simulink model "VDSAFARI"  (R2020b)
settings: Solver=VariableStepAuto  StartTime=0.0  StopTime=8.85  RelTol=1e-3
values from neighbouring files (symbols this model uses):
  AirDensity = 1.2256    [VDSUVSimlink.m]    (also in VDSafari.m)
  AirDragCoefficient = 0.45    [VDSUVSimlink.m]    (also in VDSafari.m)
  AllowedFrontLoad = 500 * g    (= 4900)    [VDSUVSimlink.m]    (also in VDSafari.m)
  CarWeight = KerbWeight + DriverWeight    (= 1745)    [VDSUVSimlink.m]    (also in VDSafari.m)
  CoefficientOfFriction = 0.9    [VDSUVSimlink.m]    (also in VDSafari.m)
  CoefficientOfRollingResistance = 0.035    [VDSUVSimlink.m]    (also in VDSafari.m)
  Equation = polyfit(EngineRadPs,EngineTorque,2)    [VDSUVSimlink.m]    (also in VDSafari.m)
  FinalDrive = 3.75    [VDSUVSimlink.m]    (also in VDSafari.m)
  FrontalArea = 3.138    [VDSUVSimlink.m]    (also in VDSafari.m)
  FrontWheelRadius = 0.369    [VDSUVSimlink.m]    (also in VDSafari.m)
  g = 9.8    [VDSUVSimlink.m]    (also in VDSafari.m)
  GearNo = Gears(1,1)    [VDSUVSimlink.m]    (also in VDSafari.m = 6)
  Gears = [1 3.96 ; 2 2.210 ; 3 1.422 ; 4 1 ; 5 0.779 ; 6 0.710]    [VDSUVSimlink.m]    (also in VDSafari.m)
  Height = 0.800    (= 0.8)    [VDSUVSimlink.m]    (also in VDSafari.m)
  MaximumEngineRPM = 3600    [VDSUVSimlink.m]    (also in VDSafari.m)
  MaximumGears = 6    [VDSUVSimlink.m]    (also in VDSafari.m)
  MinimumEngineRPM = 1200    [VDSUVSimlink.m]    (also in VDSafari.m)
  StaticFrontLoad = 0.64 *CarWeight*g    (= 10944.64)    [VDSUVSimlink.m]    (also in VDSafari.m)
  Wheelbase = 2.741    [VDSUVSimlink.m]    (also in VDSafari.m)
libraries: simulink x1
settings Model: Creator=dinesh  LastModifiedBy=dinesh

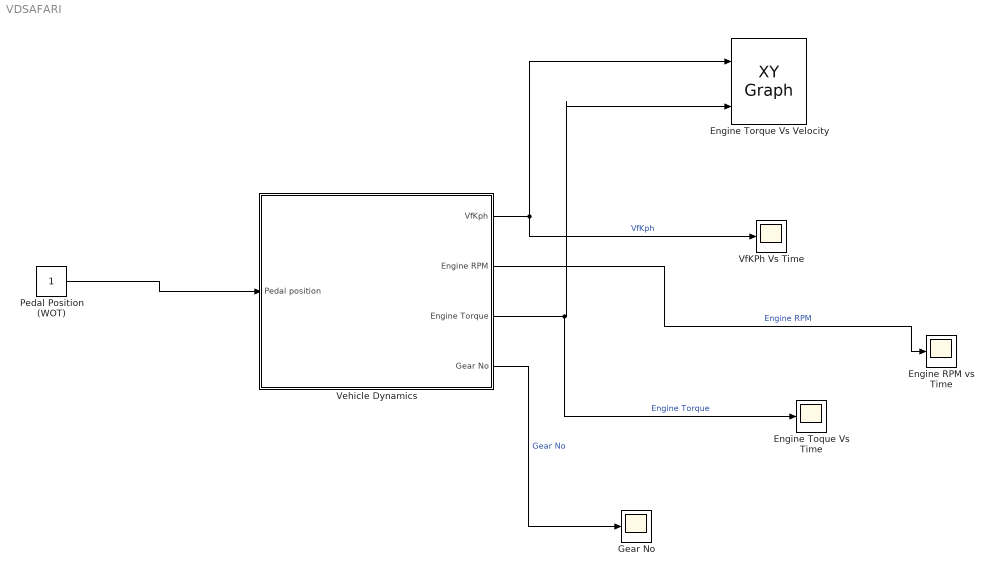
== system VDSAFARI ==
  Engine RPM vs Time : Scope
  Engine Toque Vs Time : Scope
  Engine Torque Vs Velocity : simulink/Sinks/XY Graph  xmin=0  xmax=150  ymin=0  ymax=400  st=-1
  Gear No : Scope
  Pedal Position (WOT) : Constant
  Vehicle Dynamics : Subsystem
  VfKPh Vs Time : Scope
  wires:
  Pedal Position (WOT)/1 -> Vehicle Dynamics/1(Pedal position)
  Vehicle Dynamics/3(Engine Torque) -> Engine Toque Vs Time/1, Engine Torque Vs Velocity/2  "Engine Torque"
  Vehicle Dynamics/1(VfKph) -> VfKPh Vs Time/1, Engine Torque Vs Velocity/1  "VfKph"
  Vehicle Dynamics/4(Gear No) -> Gear No/1  "Gear No"
  Vehicle Dynamics/2(Engine RPM) -> Engine RPM vs Time/1  "Engine RPM"

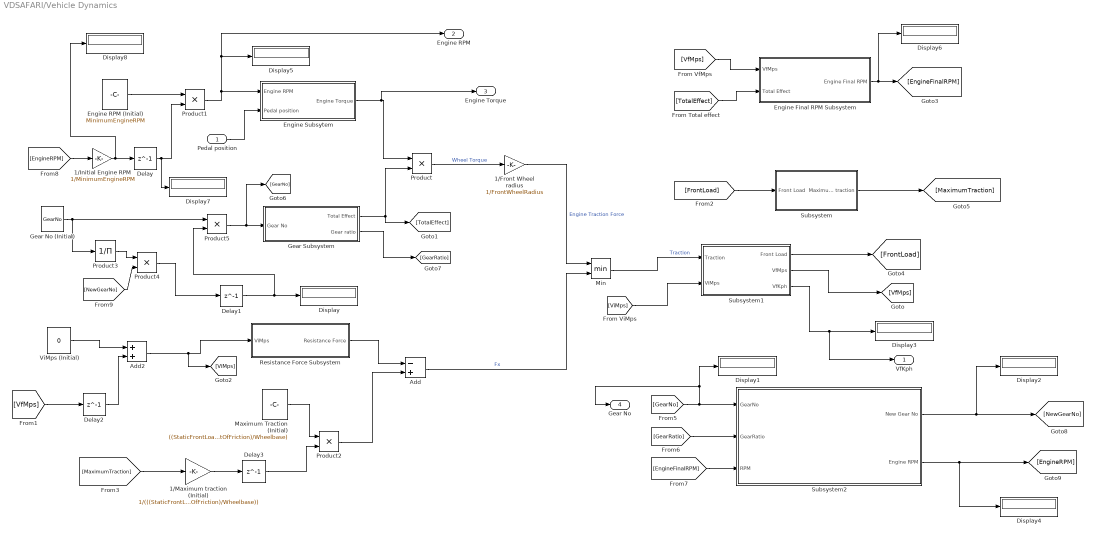
== system VDSAFARI/Vehicle Dynamics ==
  Pedal position : Inport
  1/Front Wheel radius : Gain  Gain=1/FrontWheelRadius
  1/Initial Engine RPM : Gain  Gain=1/MinimumEngineRPM
  1/Maximum traction (Initial) : Gain  Gain=1/(((StaticFrontLoad*CoefficientOfFriction))/(1+(Height*CoefficientOfFriction)/Wheelbase))
  Add : Sum  Inputs=-+
  Add2 : Sum
  Delay : Delay  DelayLength=1  InitialCondition=1  SampleTime=0.001
  Delay1 : Delay  DelayLength=1  InitialCondition=1  SampleTime=0.001
  Delay2 : Delay  DelayLength=1  InitialCondition=0  SampleTime=0.001
  Delay3 : Delay  DelayLength=1  InitialCondition=1  SampleTime=0.001
  Display{,1..8} (9 alike) : Display
  Engine Final RPM Subsystem : Subsystem
  Engine RPM (Initial) : Constant  Value=MinimumEngineRPM
  Engine Subsytem : Subsystem
  Gear No (Initial) : Constant  Value=GearNo
  Gear Subsystem : Subsystem
  Maximum Traction (Initial) : Constant  Value=((StaticFrontLoad*CoefficientOfFriction))/(1+(Height*CoefficientOfFriction)/Wheelbase)
  Min : MinMax  Inputs=2
  Product{,1..2,4..5} (5 alike) : Product
  Product3 : Product  Inputs=/
  Resistance Force Subsystem : Subsystem
  Subsystem : Subsystem
  Subsystem1 : Subsystem
  Subsystem2 : Subsystem
  ViMps (Initial) : Constant  Value=0
  VfKph : Outport
  Engine RPM : Outport  Port=2
  Engine Torque : Outport  Port=3
  Gear No : Outport  Port=4
  wires:
  Resistance Force Subsystem/1(Resistance Force) -> Add/1
  Add/1 -> Min/2  "Fx"
  Gear No (Initial)/1 -> Product5/1, Product3/1
  Engine Subsytem/1(Engine Torque) -> Engine Torque/1, Product/1
  Gear Subsystem/1(Total Effect) -> [TotalEffect], Product/2
  Product/1 -> 1/Front Wheel radius/1  "Wheel Torque"
  1/Front Wheel radius/1 -> Min/1  "Engine Traction Force"
  [TotalEffect] -> Engine Final RPM Subsystem/2(Total Effect)
  [VfMps] -> Engine Final RPM Subsystem/1(VfMps)
  Engine Final RPM Subsystem/1(Engine Final RPM) -> Display6/1, [EngineFinalRPM]
  [EngineRPM] -> 1/Initial Engine RPM/1
  1/Initial Engine RPM/1 -> Delay/1, Display8/1
  Engine RPM (Initial)/1 -> Product1/1
  Delay/1 -> Display7/1, Product1/2
  Product1/1 -> Engine RPM/1, Display5/1, Engine Subsytem/1(Engine RPM)
  [VfMps] -> Delay2/1
  ViMps (Initial)/1 -> Add2/1
  Delay2/1 -> Add2/2
  Add2/1 -> [ViMps], Resistance Force Subsystem/1(ViMps)
  [FrontLoad] -> Subsystem/1(Front Load)
  Subsystem/1(Maximum traction) -> [MaximumTraction]
  Maximum Traction (Initial)/1 -> Product2/1
  [MaximumTraction] -> 1/Maximum traction (Initial)/1
  1/Maximum traction (Initial)/1 -> Delay3/1
  Delay3/1 -> Product2/2
  Product2/1 -> Add/2
  Min/1 -> Subsystem1/1(Traction)  "Traction"
  Subsystem1/1(Front Load) -> [FrontLoad]
  Subsystem1/2(VfMps) -> [VfMps]
  Subsystem1/3(VfKph) -> VfKph/1, Display3/1
  [ViMps] -> Subsystem1/2(ViMps)
  Pedal position/1 -> Engine Subsytem/2(Pedal position)
  Gear Subsystem/2(Gear ratio) -> [GearRatio]
  Product3/1 -> Product4/1
  [NewGearNo] -> Product4/2
  Product4/1 -> Delay1/1
  Product5/1 -> [GearNo], Gear Subsystem/1(Gear No)
  [GearNo] -> Display1/1, Gear No/1, Subsystem2/1(GearNo)
  [GearRatio] -> Subsystem2/2(GearRatio)
  [EngineFinalRPM] -> Subsystem2/3(" RPM")
  Subsystem2/1(New Gear No) -> Display2/1, [NewGearNo]
  Subsystem2/2(Engine RPM) -> Display4/1, [EngineRPM]
  Delay1/1 -> Product5/2, Display/1

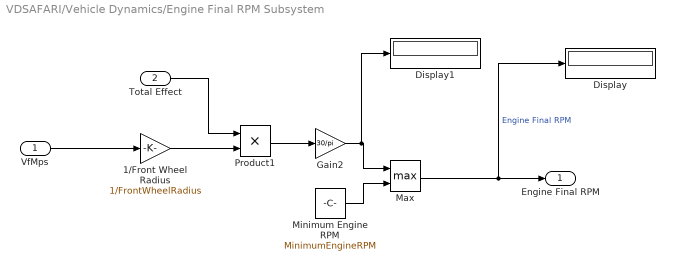
== system VDSAFARI/Vehicle Dynamics/Engine Final RPM Subsystem ==
  VfMps : Inport
  Total Effect : Inport  Port=2
  1/Front Wheel Radius : Gain  Gain=1/FrontWheelRadius
  Display : Display
  Display1 : Display
  Gain2 : Gain  Gain=30/pi
  Max : MinMax  Function=max  Inputs=2
  Minimum Engine RPM : Constant  Value=MinimumEngineRPM
  Product1 : Product
  Engine Final RPM : Outport
  wires:
  Gain2/1 -> Display1/1, Max/1
  Minimum Engine RPM/1 -> Max/2
  Max/1 -> Display/1, Engine Final RPM/1  "Engine Final RPM"
  1/Front Wheel Radius/1 -> Product1/2
  Product1/1 -> Gain2/1
  VfMps/1 -> 1/Front Wheel Radius/1
  Total Effect/1 -> Product1/1

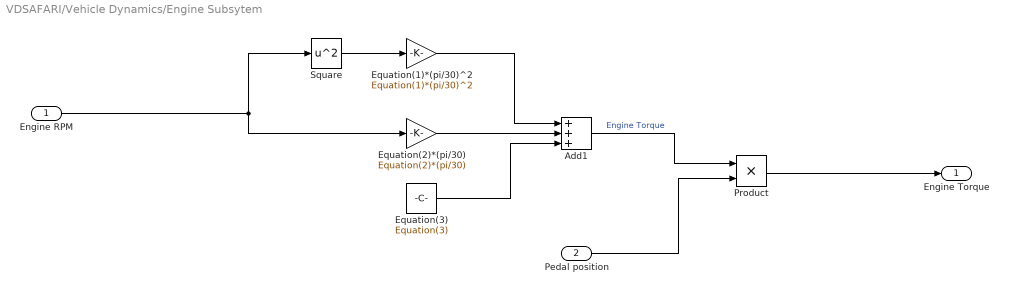
== system VDSAFARI/Vehicle Dynamics/Engine Subsytem ==
  Engine RPM : Inport
  Pedal position : Inport  Port=2
  Add1 : Sum  Inputs=+++
  "Equation(1)*(pi/30)^2 " : Gain  Gain=Equation(1)*(pi/30)^2
  Equation(2)*(pi/30) : Gain  Gain=Equation(2)*(pi/30)
  Equation(3) : Constant  Value=Equation(3)
  Product : Product
  Square : Math  Operator=square  SaturateOnIntegerOverflow=on
  Engine Torque : Outport
  wires:
  Equation(2)*(pi/30)/1 -> Add1/2
  Equation(3)/1 -> Add1/3
  Square/1 -> "Equation(1)*(pi/30)^2 "/1
  "Equation(1)*(pi/30)^2 "/1 -> Add1/1
  Engine RPM/1 -> Square/1, Equation(2)*(pi/30)/1
  Add1/1 -> Product/1  "Engine Torque"
  Pedal position/1 -> Product/2
  Product/1 -> Engine Torque/1

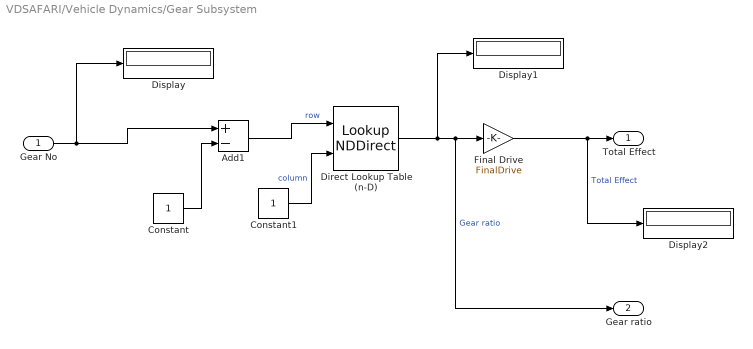
== system VDSAFARI/Vehicle Dynamics/Gear Subsystem ==
  Gear No : Inport
  Add1 : Sum  Inputs=+-
  Constant : Constant
  Constant1 : Constant
  Direct Lookup Table (n-D) : LookupNDDirect  Table=Gears  DiagnosticForOutOfRangeInput=Error
  Display : Display
  Display1 : Display
  Display2 : Display
  Final Drive : Gain  Gain=FinalDrive
  Total Effect : Outport
  Gear ratio : Outport  Port=2
  wires:
  Add1/1 -> Direct Lookup Table (n-D)/1  "row"
  Direct Lookup Table (n-D)/1 -> Display1/1, Gear ratio/1, Final Drive/1  "Gear ratio"
  Constant1/1 -> Direct Lookup Table (n-D)/2  "column"
  Constant/1 -> Add1/2
  Final Drive/1 -> Display2/1, Total Effect/1  "Total Effect"
  Gear No/1 -> Display/1, Add1/1

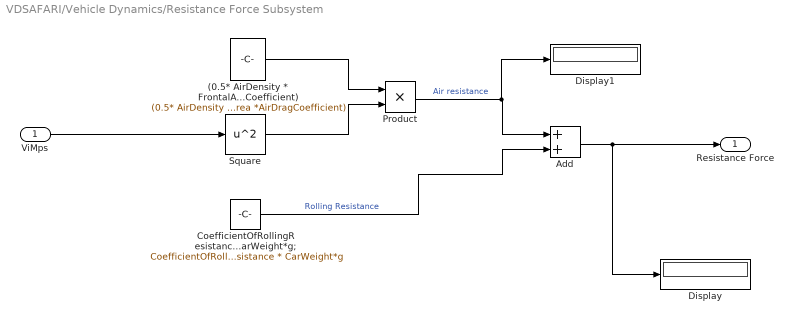
== system VDSAFARI/Vehicle Dynamics/Resistance Force Subsystem ==
  ViMps : Inport
  (0.5* AirDensity * FrontalArea * AirDragCoefficient) : Constant  Value=(0.5* AirDensity * FrontalArea *AirDragCoefficient)
  Add : Sum
  CoefficientOfRollingResistance * CarWeight*g; : Constant  Value=CoefficientOfRollingResistance * CarWeight*g
  Display : Display
  Display1 : Display
  Product : Product
  Square : Math  Operator=square  SaturateOnIntegerOverflow=on
  Resistance Force : Outport
  wires:
  Product/1 -> Display1/1, Add/1  "Air resistance"
  Add/1 -> Display/1, Resistance Force/1
  (0.5* AirDensity * FrontalArea * AirDragCoefficient)/1 -> Product/1
  Square/1 -> Product/2
  ViMps/1 -> Square/1
  CoefficientOfRollingResistance * CarWeight*g;/1 -> Add/2  "Rolling Resistance"

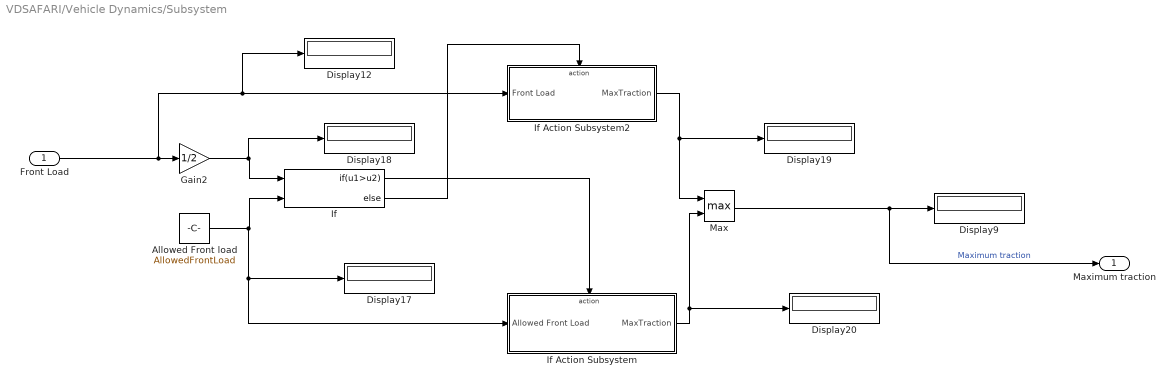
== system VDSAFARI/Vehicle Dynamics/Subsystem ==
  Front Load : Inport
  Allowed Front load : Constant  Value=AllowedFrontLoad
  Display{9,12,17..20} (6 alike) : Display
  Gain2 : Gain  Gain=1/2
  If : If  NumInputs=2  IfExpression=u1>u2
  If Action Subsystem : Subsystem  TreatAsAtomicUnit=on
  If Action Subsystem2 : Subsystem  TreatAsAtomicUnit=on
  Max : MinMax  Function=max  Inputs=2
  Maximum traction : Outport
  wires:
  If/1 -> If Action Subsystem/Action
  If/2 -> If Action Subsystem2/Action
  If Action Subsystem2/1(MaxTraction) -> Display19/1, Max/1
  Max/1 -> Maximum traction/1, Display9/1  "Maximum traction"
  Front Load/1 -> Display12/1, If Action Subsystem2/1(Front Load), Gain2/1
  Allowed Front load/1 -> Display17/1, If Action Subsystem/1(Allowed Front Load), If/2
  If Action Subsystem/1(MaxTraction) -> Max/2, Display20/1
  Gain2/1 -> Display18/1, If/1

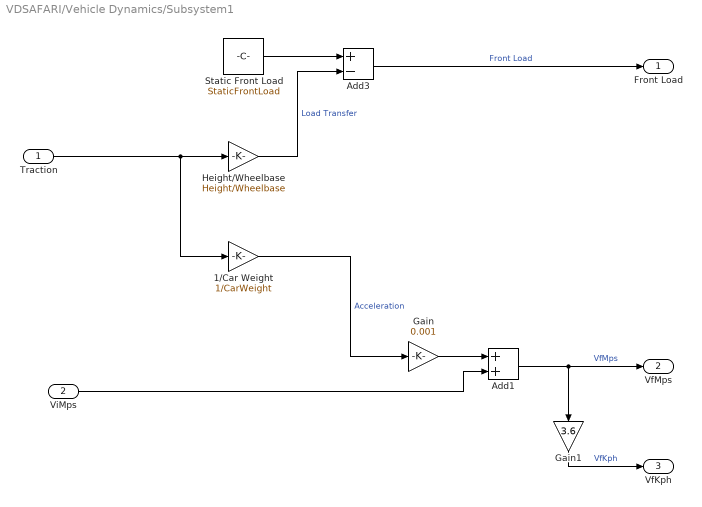
== system VDSAFARI/Vehicle Dynamics/Subsystem1 ==
  Traction : Inport
  ViMps : Inport  Port=2
  1/Car Weight : Gain  Gain=1/CarWeight
  Add1 : Sum
  Add3 : Sum  Inputs=+-
  Gain : Gain  Gain=0.001
  Gain1 : Gain  Gain=3.6
  Height/Wheelbase : Gain  Gain=Height/Wheelbase
  Static Front Load : Constant  Value=StaticFrontLoad
  Front Load : Outport
  VfMps : Outport  Port=2
  VfKph : Outport  Port=3
  wires:
  Height/Wheelbase/1 -> Add3/2  "Load Transfer"
  Gain1/1 -> VfKph/1  "VfKph"
  Add1/1 -> VfMps/1, Gain1/1  "VfMps"
  Add3/1 -> Front Load/1  "Front Load"
  Static Front Load/1 -> Add3/1
  Traction/1 -> 1/Car Weight/1, Height/Wheelbase/1
  Gain/1 -> Add1/1
  1/Car Weight/1 -> Gain/1  "Acceleration"
  ViMps/1 -> Add1/2

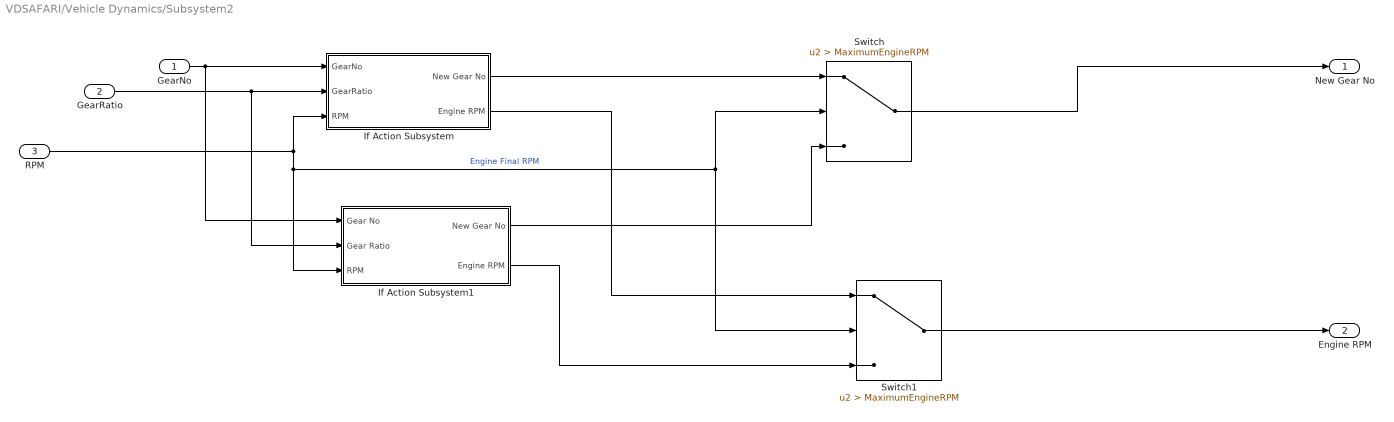
== system VDSAFARI/Vehicle Dynamics/Subsystem2 ==
  GearNo : Inport
  GearRatio : Inport  Port=2
  " RPM" : Inport  Port=3
  If Action Subsystem : Subsystem  TreatAsAtomicUnit=on
  If Action Subsystem1 : Subsystem  TreatAsAtomicUnit=on
  Switch : Switch  Criteria=u2 > Threshold  Threshold=MaximumEngineRPM
  Switch1 : Switch  Criteria=u2 > Threshold  Threshold=MaximumEngineRPM
  New Gear No : Outport
  Engine RPM : Outport  Port=2
  wires:
  If Action Subsystem1/1(New Gear No) -> Switch/3
  Switch1/1 -> Engine RPM/1
  Switch/1 -> New Gear No/1
  " RPM"/1 -> Switch/2, Switch1/2, If Action Subsystem1/3(RPM), If Action Subsystem/3(" RPM")  "Engine Final RPM"
  If Action Subsystem/1(New Gear No) -> Switch/1
  GearNo/1 -> If Action Subsystem1/1(Gear No), If Action Subsystem/1(GearNo)
  GearRatio/1 -> If Action Subsystem1/2(Gear Ratio), If Action Subsystem/2(GearRatio)
  If Action Subsystem/2(Engine RPM) -> Switch1/1
  If Action Subsystem1/2(Engine RPM) -> Switch1/3

== system VDSAFARI/Vehicle Dynamics/Subsystem/If Action Subsystem ==
  Allowed Front Load : Inport
  Action Port : ActionPort  ActionPortLabel=if(u1>u2)
  Gain : Gain  Gain=2
  mu : Gain  Gain=CoefficientOfFriction
  MaxTraction : Outport
  wires:
  Allowed Front Load/1 -> Gain/1
  Gain/1 -> mu/1
  mu/1 -> MaxTraction/1

== system VDSAFARI/Vehicle Dynamics/Subsystem/If Action Subsystem2 ==
  Front Load : Inport
  Action Port : ActionPort  ActionPortLabel=else
  Display : Display
  Display1 : Display
  mu : Gain  Gain=CoefficientOfFriction
  MaxTraction : Outport
  wires:
  Front Load/1 -> Display/1, mu/1
  mu/1 -> Display1/1, MaxTraction/1

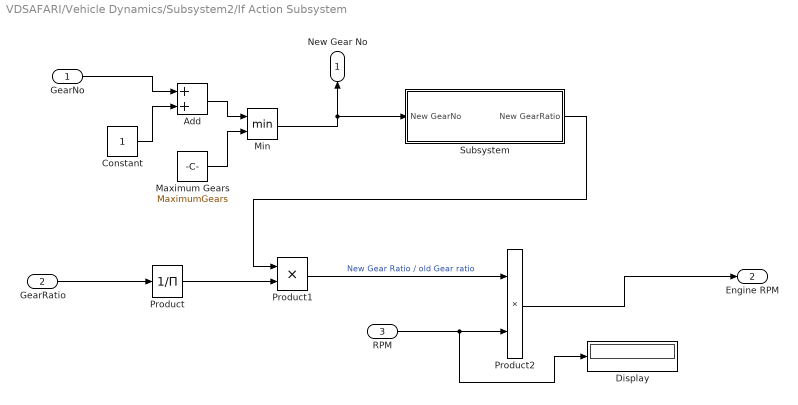
== system VDSAFARI/Vehicle Dynamics/Subsystem2/If Action Subsystem ==
  GearNo : Inport
  GearRatio : Inport  Port=2
  " RPM" : Inport  Port=3
  Add : Sum
  Constant : Constant
  Display : Display
  Maximum Gears : Constant  Value=MaximumGears
  Min : MinMax  Inputs=2
  Product : Product  Inputs=/
  Product1 : Product
  Product2 : Product
  Subsystem : Subsystem
  New Gear No : Outport
  Engine RPM : Outport  Port=2
  wires:
  GearNo/1 -> Add/1
  Constant/1 -> Add/2
  Add/1 -> Min/1
  Maximum Gears/1 -> Min/2
  Min/1 -> New Gear No/1, Subsystem/1(New GearNo)
  GearRatio/1 -> Product/1
  Product/1 -> Product1/2
  Subsystem/1(New GearRatio) -> Product1/1
  " RPM"/1 -> Display/1, Product2/2
  Product1/1 -> Product2/1  "New Gear Ratio / old Gear ratio"
  Product2/1 -> Engine RPM/1

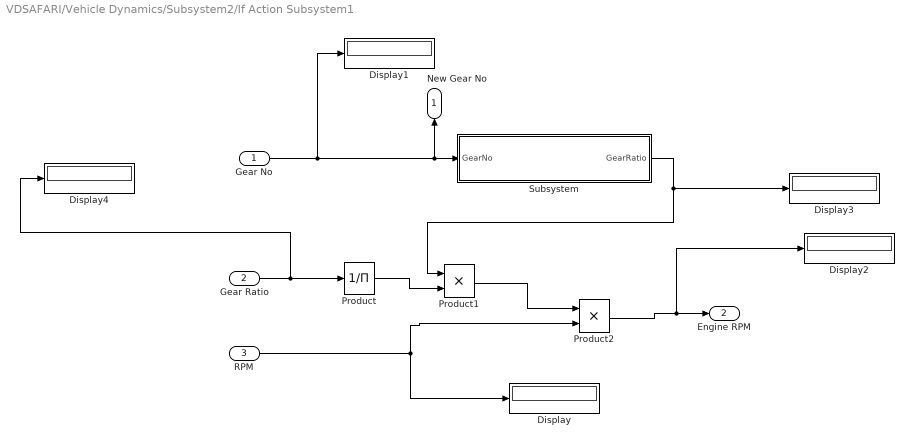
== system VDSAFARI/Vehicle Dynamics/Subsystem2/If Action Subsystem1 ==
  Gear No : Inport
  Gear Ratio : Inport  Port=2
  RPM : Inport  Port=3
  Display{,1..4} (5 alike) : Display
  Product : Product  Inputs=/
  Product1 : Product
  Product2 : Product
  Subsystem : Subsystem
  New Gear No : Outport
  Engine RPM : Outport  Port=2
  wires:
  Gear No/1 -> Display1/1, New Gear No/1, Subsystem/1(GearNo)
  Gear Ratio/1 -> Display4/1, Product/1
  Product/1 -> Product1/2
  Subsystem/1(GearRatio) -> Display3/1, Product1/1
  Product1/1 -> Product2/1
  RPM/1 -> Product2/2, Display/1
  Product2/1 -> Display2/1, Engine RPM/1

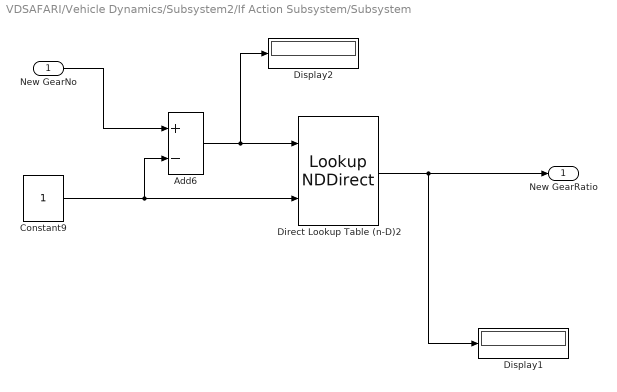
== system VDSAFARI/Vehicle Dynamics/Subsystem2/If Action Subsystem/Subsystem ==
  New GearNo : Inport
  Add6 : Sum  Inputs=+-
  Constant9 : Constant
  Direct Lookup Table (n-D)2 : LookupNDDirect  Table=Gears  DiagnosticForOutOfRangeInput=Error
  Display1 : Display
  Display2 : Display
  New GearRatio : Outport
  wires:
  Constant9/1 -> Direct Lookup Table (n-D)2/2, Add6/2
  Add6/1 -> Display2/1, Direct Lookup Table (n-D)2/1
  New GearNo/1 -> Add6/1
  Direct Lookup Table (n-D)2/1 -> Display1/1, New GearRatio/1

== system VDSAFARI/Vehicle Dynamics/Subsystem2/If Action Subsystem1/Subsystem ==
  GearNo : Inport
  Add6 : Sum  Inputs=+-
  Constant9 : Constant
  Direct Lookup Table (n-D)2 : LookupNDDirect  Table=Gears  DiagnosticForOutOfRangeInput=Error
  Display1 : Display
  Display2 : Display
  GearRatio : Outport
  wires:
  Constant9/1 -> Direct Lookup Table (n-D)2/2, Add6/2
  Add6/1 -> Display2/1, Direct Lookup Table (n-D)2/1
  GearNo/1 -> Add6/1
  Direct Lookup Table (n-D)2/1 -> Display1/1, GearRatio/1
